simulink model "SimulinkReduction"  (R2023a)
settings: Solver=VariableStepAuto  StartTime=0.0  StopTime=10.0  RelTol=1e-3
values from neighbouring files (symbols this model uses):
  c1 = 250    [VibReduction.m]
  k1 = h * myODE(ti, zi)'    [VibReduction.m]
  k2 = h * myODE(ti + h/2, zi + k1/2)'    [VibReduction.m]
  l1 = 0.23    [VibReduction.m]
  l2 = 0.17    [VibReduction.m]
  l3 = 0.14    [VibReduction.m]
settings Model: Creator=pendy  LastModifiedBy=pendy

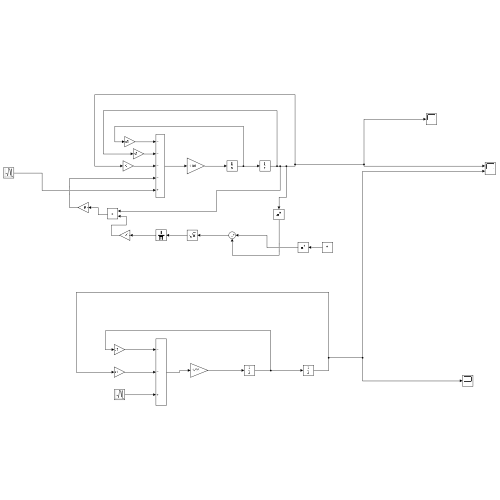
[thumbnail: Simulink's stored preview of the top-level diagram]
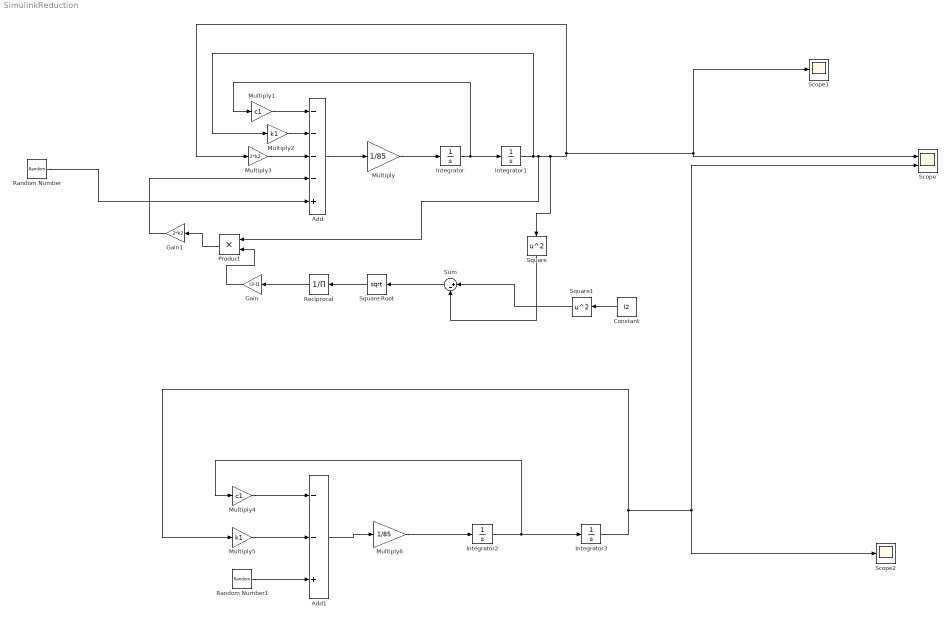
== system SimulinkReduction ==
  Add : Sum  Inputs=----+
  Add1 : Sum  Inputs=--+
  Constant : Constant  Value=l2
  Gain : Gain  Gain=l3-l1
  Gain1 : Gain  Gain=2*k2
  Integrator{,1..3} (4 alike) : Integrator
  Multiply : Gain  Gain=1/85
  Multiply1 : Gain  Gain=c1
  Multiply2 : Gain  Gain=k1
  Multiply3 : Gain  Gain=2*k2
  Multiply4 : Gain  Gain=c1
  Multiply5 : Gain  Gain=k1
  Multiply6 : Gain  Gain=1/85
  Product : Product
  Random Number : RandomNumber  SampleTime=0.1
  Random Number1 : RandomNumber  SampleTime=0.1
  Reciprocal : Product  Inputs=/
  Scope : Scope  NumInputPorts=2
  Scope1 : Scope
  Scope2 : Scope
  Square : Math  Operator=square
  Square Root : Sqrt
  Square1 : Math  Operator=square
  Sum : Sum  Inputs=|+-
  wires:
  Integrator/1 -> Multiply1/1, Integrator1/1
  Integrator1/1 -> Multiply2/1, Product/1, Square/1, Multiply3/1, Scope1/1, Scope/1
  Add/1 -> Multiply/1
  Multiply/1 -> Integrator/1
  Multiply1/1 -> Add/1
  Multiply2/1 -> Add/2
  Multiply3/1 -> Add/3
  Random Number/1 -> Add/5
  Constant/1 -> Square1/1
  Square1/1 -> Sum/1
  Square/1 -> Sum/2
  Sum/1 -> Square Root/1
  Square Root/1 -> Reciprocal/1
  Reciprocal/1 -> Gain/1
  Gain/1 -> Product/2
  Product/1 -> Gain1/1
  Gain1/1 -> Add/4
  Multiply4/1 -> Add1/1
  Multiply5/1 -> Add1/2
  Random Number1/1 -> Add1/3
  Add1/1 -> Multiply6/1
  Multiply6/1 -> Integrator2/1
  Integrator2/1 -> Multiply4/1, Integrator3/1
  Integrator3/1 -> Multiply5/1, Scope2/1, Scope/2
